simulink model "QPSK_ModulatorModel"  (R2023b)
settings: Solver=VariableStepAuto  StartTime=0.0  StopTime=10.0  RelTol=1e-3
libraries: commrandsrc3 x2, commdigbbndpm3 x2, commfilt2 x2
settings Model: Creator=judyh  LastModifiedBy=judyh

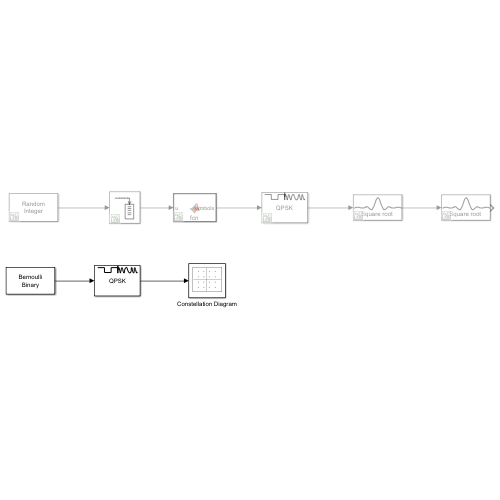
[thumbnail: Simulink's stored preview of the top-level diagram]
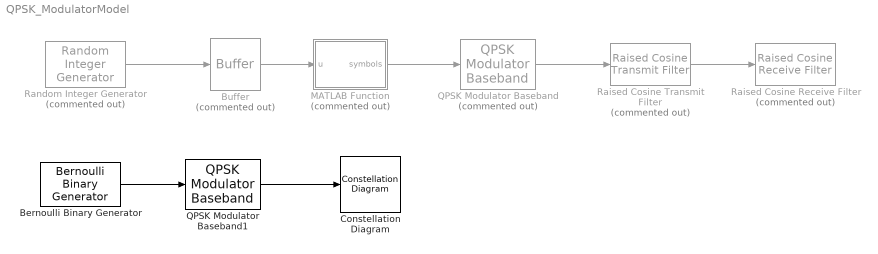
== system QPSK_ModulatorModel ==
  Bernoulli Binary Generator : commrandsrc3/Bernoulli Binary Generator  ProbabilityOfZero=0.5  SeedSource=Auto  Seed=0  SampleTime=1  SamplesPerFrame=1  OutputDataType=double  SimulateUsing=Interpreted execution
  Buffer : Buffer  Commented=on  N=10  OutputFrames=off
  Constellation Diagram : ConstellationDiagram  WindowPosition=[255.000000,117.000000,600.000000,600.000000,]  ScopeFrameLocation=window
  MATLAB Function : MATLAB Function  Commented=on  TreatAsAtomicUnit=on
  QPSK Modulator Baseband : commdigbbndpm3/QPSK Modulator Baseband  Commented=on  InType=Integer  Enc=Gray  Ph=pi/4  outDtype=double  outWordLen=16  outUDDataType=sfix(16)  outFracLenMode=Best precision  outFracLen=15  outDataTypeStr=double  outLastDataTypeStr=double
  QPSK Modulator Baseband1 : commdigbbndpm3/QPSK Modulator Baseband  InType=Integer  Enc=Gray  Ph=pi/4  outDtype=double  outWordLen=16  outUDDataType=sfix(16)  outFracLenMode=Best precision  outFracLen=15  outDataTypeStr=double  outLastDataTypeStr=double
  Raised Cosine Receive Filter : commfilt2/Raised Cosine Receive Filter  Commented=on  filtType=Square root  R=0.35  filtSpan=4  N=3  downFactor=1  downOffset=0  filterGain=1  InputProcessing=Columns as channels (frame based)  RateOptions=Enforce single-rate processing  framing=Mute  checkCoeff=off  variableName=rcRxFilt  currentFiltSpan=10  D=5  inputOffset=0  sampMode=Mute  saveAsFlag=0  rateMode=Downsampling  checkGain=Normalized  launchFVT=on  roundingMode=Floor  overflowMode=off  coeffDataTypeStr=Inherit: Same word length as input  coeffMin=[]  coeffMax=[]  coeffLastDataTypeStr=Inherit: Same word length as input  accumDataTypeStr=Inherit: Same as product output  accumLastDataTypeStr=Inherit: Same as product output  outputDataTypeStr=Inherit: Same as accumulator  outputMin=[]  outputMax=[]  outputLastDataTypeStr=Inherit: Same as accumulator
  Raised Cosine Transmit Filter : commfilt2/Raised Cosine Transmit Filter  Commented=on  filtType=Square root  R=0.35  filtSpan=4  N=3  filterGain=1  InputProcessing=Columns as channels (frame based)  RateOptions=Enforce single-rate processing  framing=Mute  checkCoeff=off  variableName=rcTxFilt  checkGain=Normalized  sampMode=Mute  saveAsFlag=0  currentFiltSpan=10  D=(10)/2  launchFVT=on  roundingMode=Floor  overflowMode=off  coeffDataTypeStr=Inherit: Same word length as input  coeffMin=[]  coeffMax=[]  coeffLastDataTypeStr=Inherit: Same word length as input  outputDataTypeStr=Inherit: Same as accumulator  outputMin=[]  outputMax=[]  outputLastDataTypeStr=Inherit: Same as accumulator
  Random Integer Generator : commrandsrc3/Random Integer Generator  Commented=on  SetSize=4  SeedSource=Auto  Seed=0  SampleTime=1e-6  SamplesPerFrame=1  OutputDataType=double  SimulateUsing=Interpreted execution
  wires:
  QPSK Modulator Baseband/1 -> Raised Cosine Transmit Filter/1
  MATLAB Function/1(symbols) -> QPSK Modulator Baseband/1
  Raised Cosine Transmit Filter/1 -> Raised Cosine Receive Filter/1
  Buffer/1 -> MATLAB Function/1(u)
  Random Integer Generator/1 -> Buffer/1
  QPSK Modulator Baseband1/1 -> Constellation Diagram/1
  Bernoulli Binary Generator/1 -> QPSK Modulator Baseband1/1

== matlab function QPSK_ModulatorModel/MATLAB Function ==
  data: u input; symbols output
function symbols = fcn(u)
    N = length(u);
    pairs = reshape(u, 2, N/2)';  % Nx2 matrix of bits
    symbols = pairs(:,1)*2 + pairs(:,2);  % Convert pairs to decimal symbols
end
